simulink model "MPC_Test"  (R2021a)
settings: Solver=FixedStepAuto  StartTime=0.0  StopTime=3  FixedStep=0.01  RelTol=1e-3
settings Model: Creator=randolf  LastModifiedBy=randolf

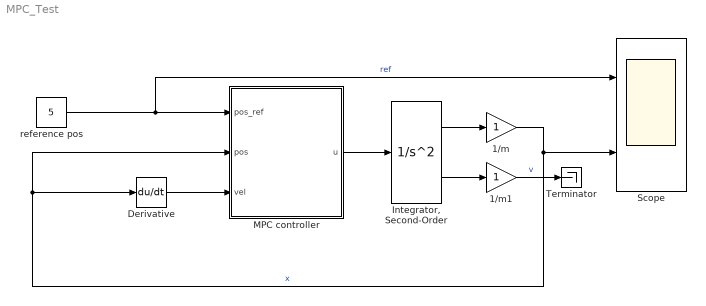
== system MPC_Test ==
  1/m : Gain
  1/m1 : Gain
  Derivative : Derivative
  "Integrator, Second-Order" : SecondOrderIntegrator
  MPC controller : MATLAB Function  TreatAsAtomicUnit=on
  Scope : Scope  NumInputPorts=2
  Terminator : Terminator
  reference pos : Constant  Value=5
  wires:
  reference pos/1 -> Scope/1, MPC controller/1(pos_ref)  "ref"
  MPC controller/1(u) -> "Integrator, Second-Order"/1
  "Integrator, Second-Order"/1 -> 1/m/1
  1/m/1 -> MPC controller/2(pos), Derivative/1, Scope/2  "x"
  Derivative/1 -> MPC controller/3(vel)
  "Integrator, Second-Order"/2 -> 1/m1/1
  1/m1/1 -> Terminator/1  "v"

== matlab function MPC_Test/MPC controller ==
  data: pos_ref input; u output; pos input; vel input
function u = MPCController(pos_ref, pos, vel)
    m = 1.05;
    T = 0.01;
    p = 45;
    Q = 10*eye(2*p);
    W = 0.0001*eye(p);
    umax = 100;
    Rk = zeros(2*p, 1);
    Rk(1:2:end) = pos_ref;
    Rk(2:2:end) = vel;
    
    xk    = [pos;vel];    %xk
    A_    = [1 T;0 1];
    B_    = [0;T/m];   
    
    psi   = zeros(2*p,2); %psi
    for i=1:1:p
        psi(i*2-1:i*2,1:2)=A_^i;
    end
    theta = zeros(2*p,p);     %theta
    for i=1:1:p
        for j=1:1:i
            theta(i*2-1:i*2,j)=A_^(i-j)*B_;
        end
    end
    E = psi*xk-Rk;            %E
    H = 2*(theta'*Q*theta+W); %H
    f = (2*E'*Q*theta)';      %f
    
    coder.extrinsic('quadprog');
    Uk=quadprog(H,f,[],[],[],[],-umax,umax);

    u = 0.0;
    u = Uk(1);  
end
